simulink model "Platoon_Event"  (R2020a)
settings: Solver=VariableStepAuto  StartTime=0.0  StopTime=100  RelTol=1e-3
undefined symbols (not defined in the file): Vehicle1
libraries: vrlib x3, simulink x2, mpcadaslib x1
settings Model: EnablePacing=on  PacingRate=100  Creator=Mustafa  LastModifiedBy=Mustafa
settings SFSimCC: CustomCodeUndefinedFunction=UseInterfaceOnly

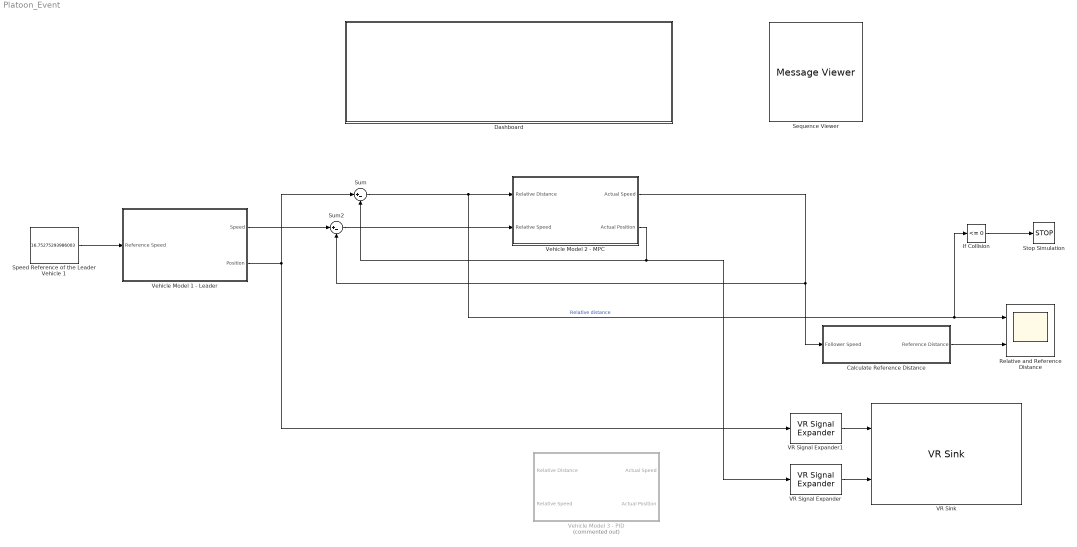
== system Platoon_Event ==
  Calculate Reference Distance : Subsystem
  Dashboard : Subsystem
  If Collision : simulink/Logic and Bit Operations/Compare To Constant  relop=<=  const=0  OutDataTypeStr=boolean
  Relative and Reference Distance : Scope  NumInputPorts=2
  Sequence Viewer : MessageViewer
  Speed Reference of the Leader Vehicle 1 : Constant  Value=16.75275293986003
  Stop Simulation : Stop
  Sum : Sum  Inputs=|+-
  Sum2 : Sum  Inputs=|+-
  VR Signal Expander : vrlib/VR Signal Expander  outwidth=3  outidx=[3]
  VR Signal Expander1 : vrlib/VR Signal Expander  outwidth=3  outidx=[3]
  VR Sink : vrlib/VR Sink  InstantiateOnLoad=on  SampleTime=0.01  ViewEnable=on  RemoteChange=off  RemoteView=off  FieldsWritten=Car_Red.translation.3.1.1.double#Car_Blue.translation.3.1.1.double  WorldFileName=PlatoonWorld.WRL  AutoView=off  VideoDimensions=[]  AllowVariableSize=off
  Vehicle Model 1 - Leader : Subsystem  mask{PositionValue=150, SpeedValue=20}
      mask prompts: PositionValue "Initial Position"; SpeedValue "Initial Speed"
      mask TypeOptions PositionValue: initial position/Value
      mask TypeOptions SpeedValue: Speed/InitialCondition
  Vehicle Model 2 - MPC : Subsystem
  Vehicle Model 3 - PID : Subsystem  Commented=on
  wires:
  Calculate Reference Distance/1(Reference Distance) -> Relative and Reference Distance/2
  Vehicle Model 2 - MPC/1(Actual Speed) -> Sum2/2, Calculate Reference Distance/1(Follower Speed)
  Vehicle Model 1 - Leader/2(Position) -> Sum/1, VR Signal Expander1/1
  Sum/1 -> Vehicle Model 2 - MPC/1(Relative Distance), If Collision/1, Relative and Reference Distance/1  "Relative distance"
  Sum2/1 -> Vehicle Model 2 - MPC/2(Relative Speed)
  Vehicle Model 1 - Leader/1("Speed ") -> Sum2/1
  Speed Reference of the Leader Vehicle 1/1 -> Vehicle Model 1 - Leader/1(Reference Speed)
  Vehicle Model 2 - MPC/2(Actual Position) -> Sum/2, VR Signal Expander/1
  VR Signal Expander1/1 -> VR Sink/1
  VR Signal Expander/1 -> VR Sink/2
  If Collision/1 -> Stop Simulation/1

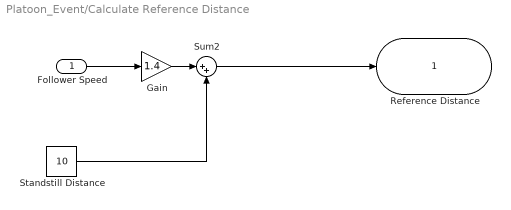
== system Platoon_Event/Calculate Reference Distance ==
  Follower Speed : Inport
  Gain : Gain  Gain=1.4
  Standstill Distance : Constant  Value=10
  Sum2 : Sum  Inputs=|++
  Reference Distance : Outport  VectorParamsAs1DForOutWhenUnconnected=off
  wires:
  Sum2/1 -> Reference Distance/1
  Gain/1 -> Sum2/1
  Follower Speed/1 -> Gain/1
  Standstill Distance/1 -> Sum2/2

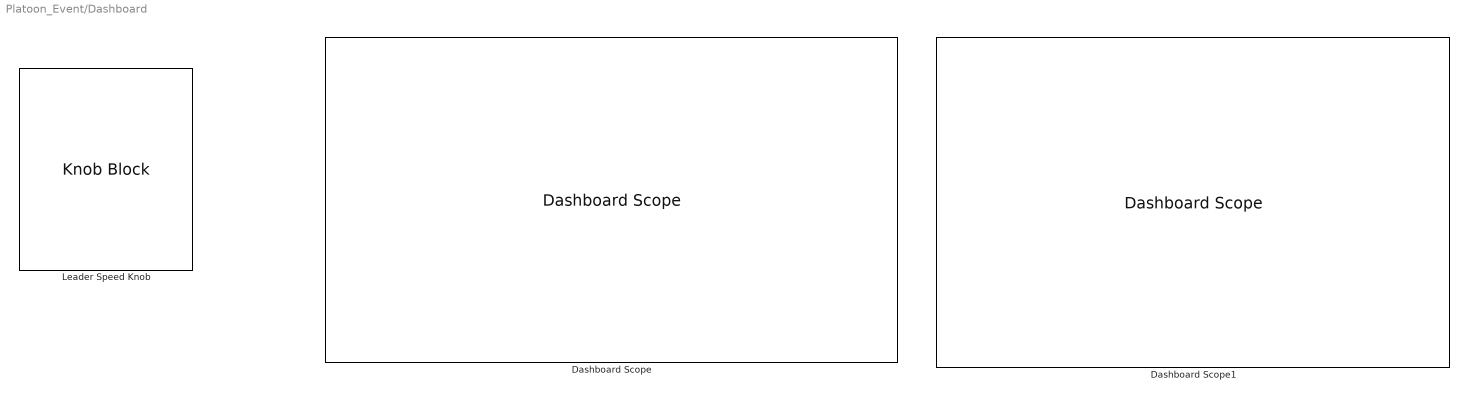
== system Platoon_Event/Dashboard ==
  Dashboard Scope : DashboardScope  Ymin=-5  Ymax=200
  Dashboard Scope1 : DashboardScope  Ymin=-5  Ymax=200
  Leader Speed Knob : KnobBlock  ScaleMax=50  TickInterval=5

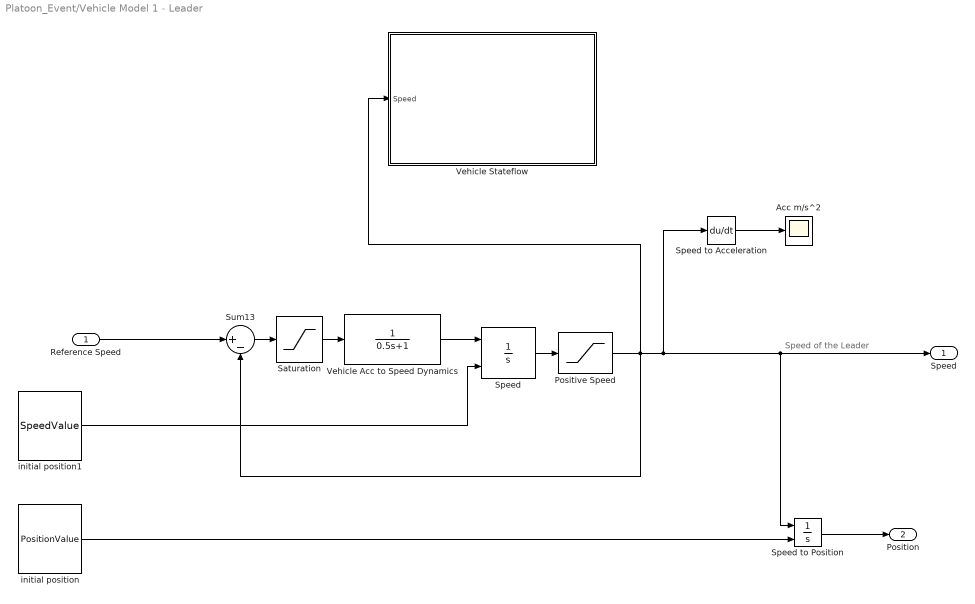
== system Platoon_Event/Vehicle Model 1 - Leader ==
  note: Speed of the Leader
  Reference Speed : Inport
  Acc m/s^2 : Scope
  Positive Speed : Saturate  UpperLimit=inf  LowerLimit=0
  Saturation : Saturate  UpperLimit=2  LowerLimit=-3
  Speed : Integrator  InitialConditionSource=external  InitialCondition=SpeedValue
  Speed to Acceleration : Derivative
  Speed to Position : Integrator  InitialConditionSource=external  InitialCondition=Vehicle1.position
  Sum13 : Sum  Inputs=|+-
  Vehicle Acc to Speed Dynamics : TransferFcn  Denominator=[0.5 1]
  Vehicle Stateflow : Stateflow chart  TreatAsAtomicUnit=on
  initial position : Constant  Value=PositionValue
  initial position1 : Constant  Value=SpeedValue
  "Speed " : Outport  VectorParamsAs1DForOutWhenUnconnected=off
  Position : Outport  Port=2  VectorParamsAs1DForOutWhenUnconnected=off
  wires:
  Speed to Acceleration/1 -> Acc m/s^2/1
  Speed to Position/1 -> Position/1
  initial position/1 -> Speed to Position/2
  Vehicle Acc to Speed Dynamics/1 -> Speed/1
  Sum13/1 -> Saturation/1
  Saturation/1 -> Vehicle Acc to Speed Dynamics/1
  Reference Speed/1 -> Sum13/1
  Positive Speed/1 -> Vehicle Stateflow/1(Speed), Speed to Position/1, "Speed "/1, Speed to Acceleration/1, Sum13/2
  initial position1/1 -> Speed/2
  Speed/1 -> Positive Speed/1

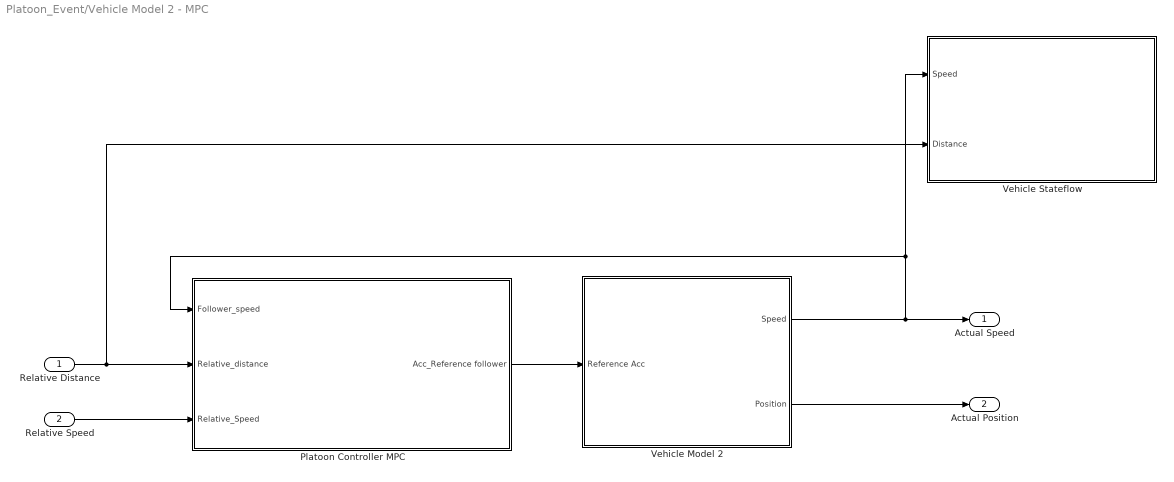
== system Platoon_Event/Vehicle Model 2 - MPC ==
  Relative Distance : Inport
  Relative Speed : Inport  Port=2
  Platoon Controller MPC : Subsystem
  Vehicle Model 2 : Subsystem  mask{PositionValue=0, SpeedValue=30}
      mask prompts: PositionValue "Initial Position"; SpeedValue "Initial Speed"
      mask TypeOptions PositionValue: initial position/Value
      mask TypeOptions SpeedValue: Speed/InitialCondition
  Vehicle Stateflow : Stateflow chart  TreatAsAtomicUnit=on
  Actual Speed : Outport  VectorParamsAs1DForOutWhenUnconnected=off
  Actual Position : Outport  Port=2  VectorParamsAs1DForOutWhenUnconnected=off
  wires:
  Vehicle Model 2/2(Position) -> Actual Position/1
  Vehicle Model 2/1("Speed ") -> Actual Speed/1, Vehicle Stateflow/1(Speed), Platoon Controller MPC/1(Follower_speed)
  Platoon Controller MPC/1(Acc_Reference follower) -> Vehicle Model 2/1(Reference Acc)
  Relative Distance/1 -> Vehicle Stateflow/2(Distance), Platoon Controller MPC/2(Relative_distance)
  Relative Speed/1 -> Platoon Controller MPC/3(Relative_Speed)

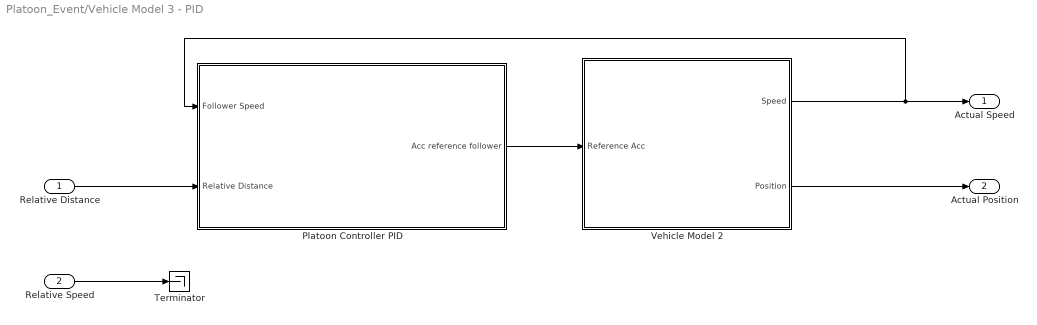
== system Platoon_Event/Vehicle Model 3 - PID ==
  Relative Distance : Inport
  Relative Speed : Inport  Port=2
  Platoon Controller PID : Subsystem
  Terminator : Terminator
  Vehicle Model 2 : Subsystem  mask{PositionValue=0, SpeedValue=30}
      mask prompts: PositionValue "Initial Position"; SpeedValue "Initial Speed"
      mask TypeOptions PositionValue: initial position/Value
      mask TypeOptions SpeedValue: Speed/InitialCondition
  Actual Speed : Outport  VectorParamsAs1DForOutWhenUnconnected=off
  Actual Position : Outport  Port=2  VectorParamsAs1DForOutWhenUnconnected=off
  wires:
  Vehicle Model 2/2(Position) -> Actual Position/1
  Vehicle Model 2/1("Speed ") -> Platoon Controller PID/1(Follower Speed), Actual Speed/1
  Platoon Controller PID/1(Acc reference follower) -> Vehicle Model 2/1(Reference Acc)
  Relative Distance/1 -> Platoon Controller PID/2(Relative Distance)
  Relative Speed/1 -> Terminator/1

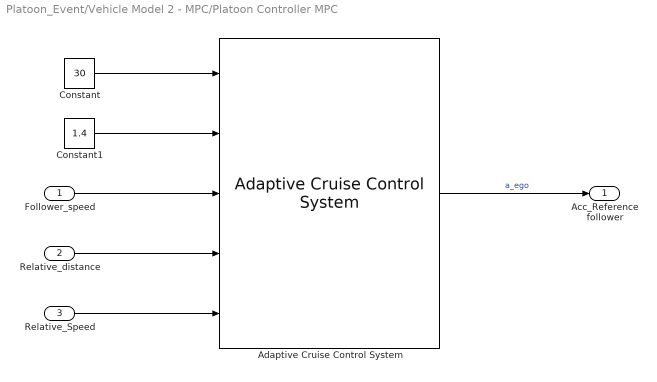
== system Platoon_Event/Vehicle Model 2 - MPC/Platoon Controller MPC ==
  Follower_speed : Inport
  Relative_distance : Inport  Port=2
  Relative_Speed : Inport  Port=3
  Adaptive Cruise Control System : mpcadaslib/Adaptive Cruise Control System  EgoModel=tf(1,[0.5,1,0])  InitialEgoVelocity=30  DefaultSpacing=10  MaxVelocity=50  MinAcceleration=-3  amin_ext=off  MaxAcceleration=2  amax_ext=off  Ts=0.1  PredictionHorizon=300  ControllerBehavior=0.800  suboptimal=off  maxiter=100  datatypeopt=double  optmode=off  trackmode=off
  Constant : Constant  Value=30
  Constant1 : Constant  Value=1.4
  Acc_Reference follower : Outport  VectorParamsAs1DForOutWhenUnconnected=off
  wires:
  Follower_speed/1 -> Adaptive Cruise Control System/3
  Relative_distance/1 -> Adaptive Cruise Control System/4
  Relative_Speed/1 -> Adaptive Cruise Control System/5
  Adaptive Cruise Control System/1 -> Acc_Reference follower/1  "a_ego"
  Constant/1 -> Adaptive Cruise Control System/1
  Constant1/1 -> Adaptive Cruise Control System/2

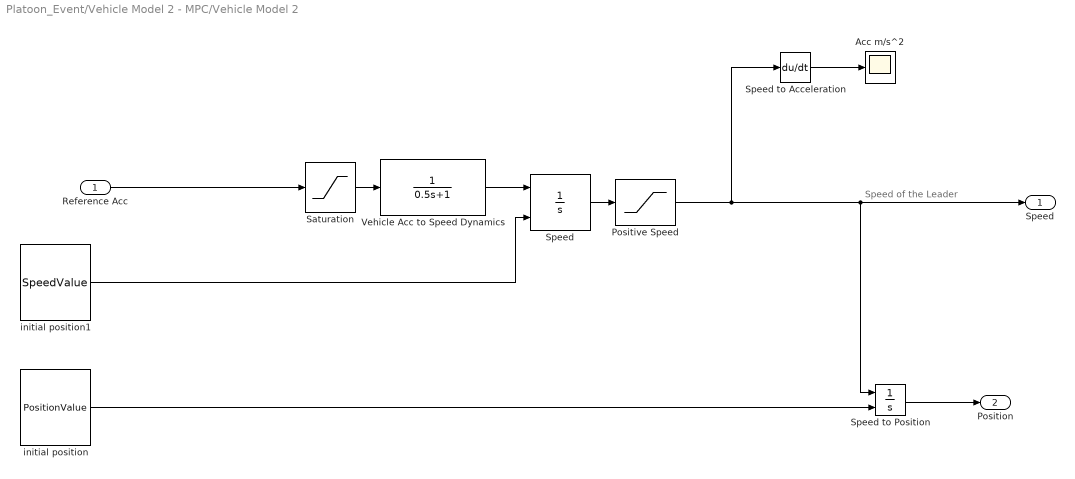
== system Platoon_Event/Vehicle Model 2 - MPC/Vehicle Model 2 ==
  note: Speed of the Leader
  Reference Acc : Inport
  Acc m/s^2 : Scope
  Positive Speed : Saturate  UpperLimit=inf  LowerLimit=0
  Saturation : Saturate  UpperLimit=2  LowerLimit=-3
  Speed : Integrator  InitialConditionSource=external  InitialCondition=SpeedValue
  Speed to Acceleration : Derivative
  Speed to Position : Integrator  InitialConditionSource=external  InitialCondition=Vehicle1.position
  Vehicle Acc to Speed Dynamics : TransferFcn  Denominator=[0.5 1]
  initial position : Constant  Value=PositionValue
  initial position1 : Constant  Value=SpeedValue
  "Speed " : Outport  VectorParamsAs1DForOutWhenUnconnected=off
  Position : Outport  Port=2  VectorParamsAs1DForOutWhenUnconnected=off
  wires:
  Speed to Acceleration/1 -> Acc m/s^2/1
  Speed to Position/1 -> Position/1
  initial position/1 -> Speed to Position/2
  Vehicle Acc to Speed Dynamics/1 -> Speed/1
  Reference Acc/1 -> Saturation/1
  Saturation/1 -> Vehicle Acc to Speed Dynamics/1
  Positive Speed/1 -> Speed to Position/1, "Speed "/1, Speed to Acceleration/1
  initial position1/1 -> Speed/2
  Speed/1 -> Positive Speed/1

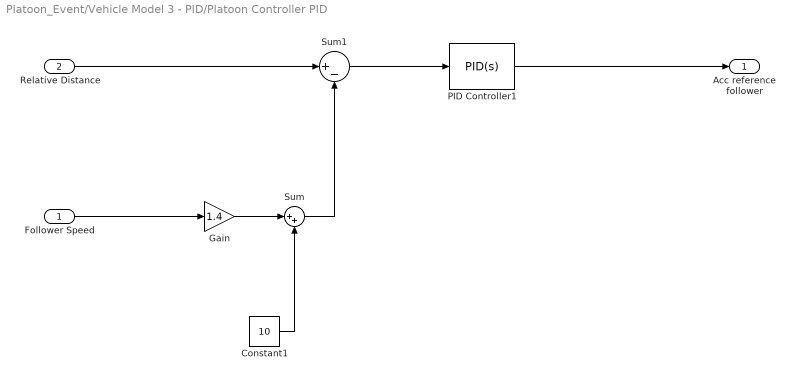
== system Platoon_Event/Vehicle Model 3 - PID/Platoon Controller PID ==
  Follower Speed : Inport
  Relative Distance : Inport  Port=2
  Constant1 : Constant  Value=10
  Gain : Gain  Gain=1.4
  PID Controller1 : simulink/Continuous/PID Controller  Controller=PID  Form=Parallel  TimeDomain=Continuous-time  UseExternalTs=off  SampleTime=0.1  IntegratorMethod=Forward Euler  FilterMethod=Forward Euler  ControllerParametersSource=internal  P=2.0341199375219  I=0.0356576460366845  D=2.08363010404189  UseFilter=on  N=233.214579742572  TunerSelectOption=Transfer Function Based (PID Tuner App)  InitialConditionSource=internal  InitialConditionForIntegrator=0  InitialConditionForFilter=0  DifferentiatorICPrevScaledInput=0  ExternalReset=none  TrackingMode=off  Kt=1  LimitOutput=on  UpperSaturationLimit=2  LowerSaturationLimit=-3  LinearizeAsGain=on  AntiWindupMode=clamping  Kb=1  POutMin=[]  POutMax=[]  IOutMin=[]  IOutMax=[]  DOutMin=[]  DOutMax=[]  NOutMin=[]  NOutMax=[]  SumOutMin=[]  SumOutMax=[]  SaturationOutMin=[]  SaturationOutMax=[]  PParamMin=[]  PParamMax=[]  IParamMin=[]  IParamMax=[]  DParamMin=[]  DParamMax=[]  NParamMin=[]  NParamMax=[]  KbParamMin=[]  KbParamMax=[]  KtParamMin=[]  KtParamMax=[]  KbOutMin=[]  KbOutMax=[]  KtOutMin=[]  KtOutMax=[]  IntegratorOutMin=[]  IntegratorOutMax=[]  FilterOutMin=[]  FilterOutMax=[]  SumI1OutMin=[]  SumI1OutMax=[]  SumI2OutMin=[]  SumI2OutMax=[]  SumI3OutMin=[]  SumI3OutMax=[]  SumI4OutMin=[]  SumI4OutMax=[]  SumDOutMin=[]  SumDOutMax=[]  DifferentiatorOutMin=[]  DifferentiatorOutMax=[]  FilterDiffOutCoefMin=[]  FilterDiffOutCoefMax=[]  ReciprocalOutMin=[]  ReciprocalOutMax=[]  SumDenOutMin=[]  SumDenOutMax=[]  SumNumOutMin=[]  SumNumOutMax=[]  DivideOutMin=[]  DivideOutMax=[]  UdiffTsProdOutMin=[]  UdiffTsProdOutMax=[]  NTsProdOutMin=[]  NTsProdOutMax=[]  UintegralTsProdOutMin=[]  UintegralTsProdOutMax=[]  UngainTsProdOutMin=[]  UngainTsProdOutMax=[]  IntegratorContinuousStateAttributes=''  IntegratorStateMustResolveToSignalObject=off  IntegratorRTWStateStorageClass=Auto  FilterContinuousStateAttributes=''  FilterStateMustResolveToSignalObject=off  FilterRTWStateStorageClass=Auto  ParallelPVariant=InternalParameters  IdealPVariant=Disabled  IVariant=InternalParameters  DVariant=InternalParameters  IntegratorVariant=Continuous  SatVariant=Enabled  AWVariant=ContClampingParallel  PCopyVariant=Disabled  TRVariant=Disabled  FdbkBlocksVariant=Forward  IdealPFdbkVariant=Disabled  SatFdbkVariant=Disabled  DerivativeFilterVariant=ContFilter  NVariant=InternalParameters  NCopyVariant=Disabled  FilterICVariant=InternalICsFilter  IntegratorICVariant=InternalICs  ExternalResetVariant=Disabled  TRSumVariant=Passthrough  SumFdbkVariant=Disabled  SumVariant=Sum_PID  TsampFilterVariant=InternalTs  TsampNgainVariant=Passthrough  TsampIntegralVariant=Passthrough
  Sum : Sum  Inputs=|++
  Sum1 : Sum  Inputs=|+-
  Acc reference follower : Outport  VectorParamsAs1DForOutWhenUnconnected=off
  wires:
  Relative Distance/1 -> Sum1/1
  Follower Speed/1 -> Gain/1
  Sum1/1 -> PID Controller1/1
  Constant1/1 -> Sum/2
  Gain/1 -> Sum/1
  Sum/1 -> Sum1/2
  PID Controller1/1 -> Acc reference follower/1

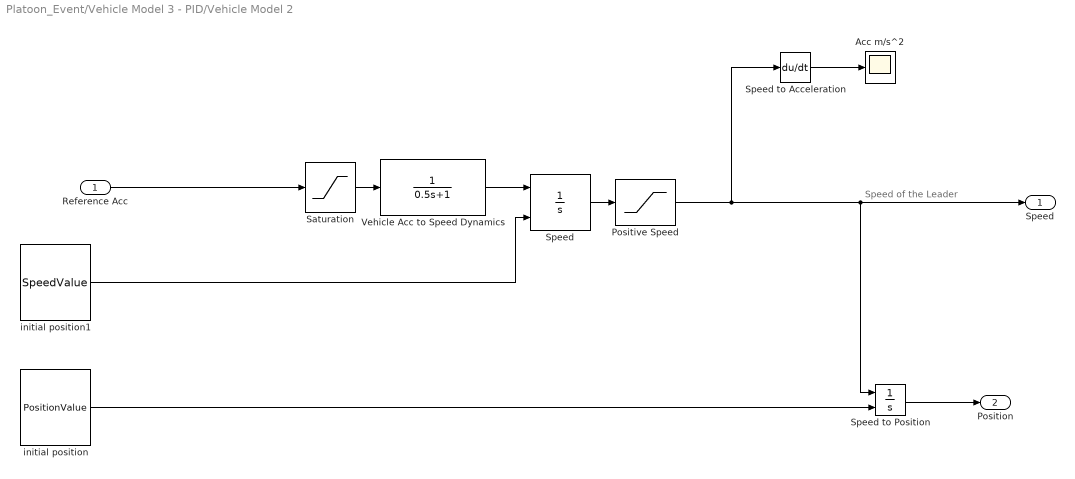
== system Platoon_Event/Vehicle Model 3 - PID/Vehicle Model 2 ==
  note: Speed of the Leader
  Reference Acc : Inport
  Acc m/s^2 : Scope
  Positive Speed : Saturate  UpperLimit=inf  LowerLimit=0
  Saturation : Saturate  UpperLimit=2  LowerLimit=-3
  Speed : Integrator  InitialConditionSource=external  InitialCondition=SpeedValue
  Speed to Acceleration : Derivative
  Speed to Position : Integrator  InitialConditionSource=external  InitialCondition=Vehicle1.position
  Vehicle Acc to Speed Dynamics : TransferFcn  Denominator=[0.5 1]
  initial position : Constant  Value=PositionValue
  initial position1 : Constant  Value=SpeedValue
  "Speed " : Outport  VectorParamsAs1DForOutWhenUnconnected=off
  Position : Outport  Port=2  VectorParamsAs1DForOutWhenUnconnected=off
  wires:
  Speed to Acceleration/1 -> Acc m/s^2/1
  Speed to Position/1 -> Position/1
  initial position/1 -> Speed to Position/2
  Vehicle Acc to Speed Dynamics/1 -> Speed/1
  Reference Acc/1 -> Saturation/1
  Saturation/1 -> Vehicle Acc to Speed Dynamics/1
  Positive Speed/1 -> Speed to Position/1, "Speed "/1, Speed to Acceleration/1
  initial position1/1 -> Speed/2
  Speed/1 -> Positive Speed/1

== stateflow chart Platoon_Event/Vehicle Model 2 - MPC/Vehicle Stateflow ==
  state VEHICLE_STOPS
  state VEHICLE_MOVING
    state SpeedSituation [parallel]
      settings: executionOrder=1
      state Slow
      state Fast
      (default) -> Slow
      Fast -> Slow : [Speed<10]
      Slow -> Fast : [Speed>10]
    state DrivingMode [parallel]
      settings: executionOrder=2
      state Close
      state Far
      (default) -> Close
      Far -> Close : [Distance<50]
      Close -> Far : [Distance>50]
  (default) -> VEHICLE_STOPS
  VEHICLE_STOPS -> VEHICLE_MOVING : [Speed>0]
  VEHICLE_MOVING -> VEHICLE_STOPS : [Speed==0]
  data: Speed input; Distance input

== stateflow chart Platoon_Event/Vehicle Model 1 - Leader/Vehicle Stateflow ==
  state VEHICLE_STOPS
  state VEHICLE_MOVING
    state Slow
    state Fast
    (default) -> Slow
    Fast -> Slow : [Speed<10]
    Slow -> Fast : [Speed>10]
  (default) -> VEHICLE_STOPS
  VEHICLE_STOPS -> VEHICLE_MOVING : [Speed>0]
  VEHICLE_MOVING -> VEHICLE_STOPS : [Speed==0]
  data: Speed input
